simulink model "ur3_simulink_ros2_ibvs_mpc"  (R2023b)
settings: Solver=ode4  StartTime=0.0  StopTime=Inf  FixedStep=0.005  RelTol=1e-3
model workspace (MAT data in the model file):
  SL_ROS_VariableLengthArrays_MaxSizes.CommonInfo.ArrayTruncateAction = 'EmitWarning'
  SL_ROS_VariableLengthArrays_MaxSizes.MsgTypeMap = containers.Map
  SL_ROS_VariableLengthArrays_MaxSizes.MsgTypeMap.serialization.keys = {'example_interfaces/Float64MultiArray'}
  SL_ROS_VariableLengthArrays_MaxSizes.MsgTypeMap.serialization.values{1}.PropertyName = 'data'
  SL_ROS_VariableLengthArrays_MaxSizes.MsgTypeMap.serialization.values{1}.DataType = 'double'
  SL_ROS_VariableLengthArrays_MaxSizes.MsgTypeMap.serialization.values{1}.MaxLength = 1
  SL_ROS_VariableLengthArrays_MaxSizes.MsgTypeMap.serialization.uniformity = 0
  SL_ROS_VariableLengthArrays_MaxSizes.MsgTypeMap.serialization.keyType = 'char'
  SL_ROS_VariableLengthArrays_MaxSizes.MsgTypeMap.serialization.valueType = 'any'
undefined symbols (not defined in the file): data, data_SL_Info
libraries: simulink x9, ros2lib x8, robotmaniplib x3, robotcorelib x2, dspinverses x1, mpclib x1
(part 1 of 2)
settings Model: SimulationMode=accelerator  Creator=81232  LastModifiedBy=Administrator
settings OptimizationCC: EnhancedBackFolding=on  PassReuseOutputArgsAs=Individual arguments  ZeroExternalMemoryAtStartup=off  ZeroInternalMemoryAtStartup=off  MaxStackSize=64  OptimizeBlockOrder=speed  DifferentSizesBufferReuse=on  OptimizationCustomize=off  EfficientTunableParamExpr=on
settings DebuggingCC: ParameterTunabilityLossMsg=error
settings ModelReferenceCC: EnableRefExpFcnMdlSchedulingChecks=on
settings SFSimCC: MATLABDynamicMemAlloc=off
settings RTWCC: Description=Embedded Coder  SystemTargetFile=ert.tlc  HardwareBoard=Robot Operating System 2 (ROS 2)  TLCOptions="-aInlineSetEventsForThisBaseRateFcn=TLC_FALSE -aSuppressMultiTaskScheduler=TLC_FALSE  -aRateBasedStepFcn=0"  TemplateMakefile=ert_default_tmf  Toolchain=Colcon Tools  TargetLang=C++
settings CodeAppCC: ForceParamTrailComments=on  IgnoreCustomStorageClasses=off  OperatorAnnotations=on  SimulinkDataObjDesc=on  SFDataObjDesc=on  InsertBlockDesc=on
settings ERTTargetCC: CodeInterfacePackaging=C++ class  RootIOFormat=Structure reference

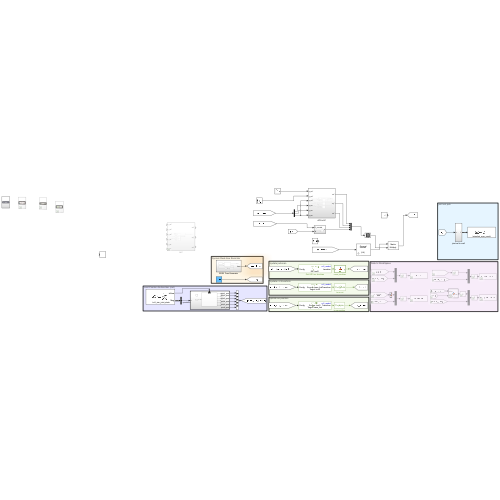
[thumbnail: Simulink's stored preview of the top-level diagram]
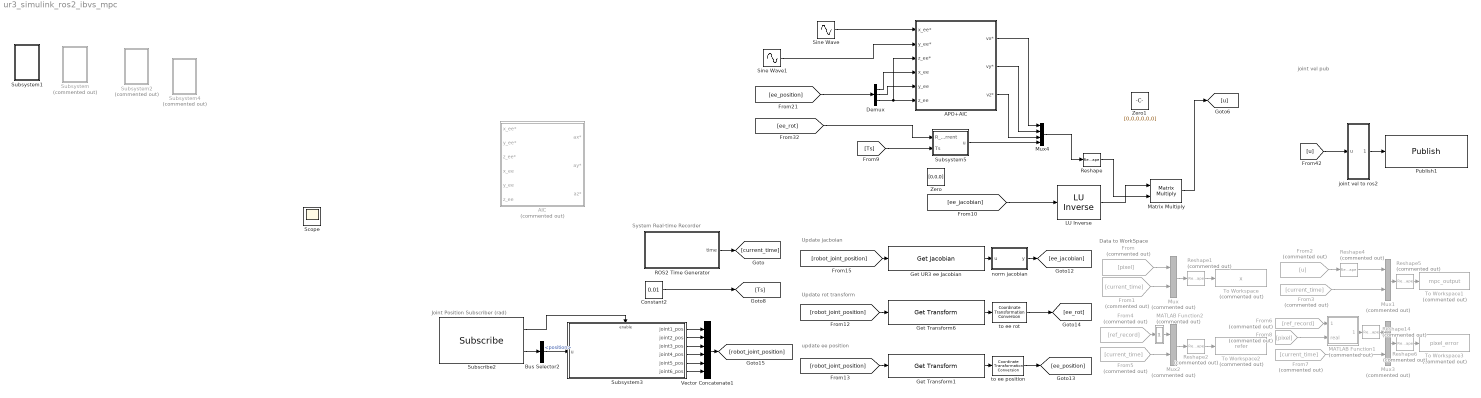
== system ur3_simulink_ros2_ibvs_mpc ==
  note: joint vel pub
  note: update ee position
  note: Update rot transform
  note: Joint Position Subscriber (rad)
  note: Data to WorkSpace
  note: System Real-time Recorder
  note: Update jacboian
  " LU Inverse" : dspinverses/ LU Inverse
  AIC : Subsystem  Commented=on
  APO+AIC : Subsystem
  Bus Selector2 : BusSelector  OutputSignals=position
  Constant2 : Constant  Value=0.01
  Demux : Demux  Outputs=3
  From : From  Commented=on  GotoTag=pixel
  From{1,3,5,7} (4 alike) : From  Commented=on  GotoTag=current_time
  From2 : From  Commented=on  GotoTag=u
  From4 : From  Commented=on  GotoTag=ref_record
  From6 : From  Commented=on  GotoTag=ref_record
  From8 : From  Commented=on  GotoTag=pixel
  Get Transform1 : robotmaniplib/Get Transform  RigidBodyTree=ur3_model  SourceBody=tool0  TargetBody=base_link  SimulateUsing=Interpreted execution
  Get Transform6 : robotmaniplib/Get Transform  RigidBodyTree=ur3_model  SourceBody=base_link  TargetBody=tool0  SimulateUsing=Interpreted execution
  Get UR3 ee Jacobian : robotmaniplib/Get Jacobian  RigidBodyTree=ur3_model  EndEffector=tool0  SimulateUsing=Interpreted execution
  MATLAB Function1 : MATLAB Function  Commented=on  TreatAsAtomicUnit=on
  MATLAB Function2 : MATLAB Function  Commented=on  TreatAsAtomicUnit=on
  Matrix Multiply : Product  Multiplication=Matrix(*)
  Mux{,1..3} (4 alike) : Mux  Commented=on  Inputs=2
  Mux4 : Mux
  Publish1 : ros2lib/Publish  topicSource=Select from ROS network  topic=/simulink_mpc_result  messageType=std_msgs/Float64MultiArray  QOSHistory=Keep last  QOSDepth=1  QOSReliability=Reliable  QOSDurability=Volatile
      settings: LibrarySourceBlock=roslib/ROS 2/Publish
  ROS2 Time Generator : Subsystem
  Reshape : Reshape  OutputDimensionality=Column vector (2-D)
  Reshape1 : Reshape  Commented=on  OutputDimensionality=Customize  OutputDimensions=[9]
  Reshape14 : Reshape  Commented=on  OutputDimensionality=Customize  OutputDimensions=[8,1]
  Reshape2 : Reshape  Commented=on  OutputDimensionality=Customize  OutputDimensions=[9]
  Reshape4 : Reshape  Commented=on  OutputDimensionality=Customize  OutputDimensions=[6,1]
  Reshape5 : Reshape  Commented=on  OutputDimensionality=Customize  OutputDimensions=[7]
  Reshape6 : Reshape  Commented=on  OutputDimensionality=Customize  OutputDimensions=[9]
  Scope : Scope
  Sine Wave : Sin  Amplitude=0.15  Bias=-0.1  Frequency=1.6  SampleTime=0
  Sine Wave1 : Sin  Amplitude=0.15  Bias=0.3  Frequency=1.6  Phase=pi/2  SampleTime=0
  Subscribe2 : ros2lib/Subscribe  topicSource=Select from ROS network  topic=/ur3_sim_joint_state  messageType=sensor_msgs/JointState  sampleTime=0.005  QOSHistory=Keep last  QOSDepth=1  QOSReliability=Reliable  QOSDurability=Volatile
  Subsystem : Subsystem  Commented=on
  Subsystem1 : Subsystem
  Subsystem2 : Subsystem  Commented=on
  Subsystem3 : Subsystem
  Subsystem4 : Subsystem  Commented=on
  Subsystem5 : Subsystem
  To Workspace : ToWorkspace  Commented=on  VariableName=x  SaveFormat=Timeseries  SampleTime=-1
  To Workspace1 : ToWorkspace  Commented=on  VariableName=mpc_output  SaveFormat=Timeseries  SampleTime=-1
  To Workspace2 : ToWorkspace  Commented=on  VariableName=refer  SaveFormat=Timeseries  SampleTime=-1
  To Workspace3 : ToWorkspace  Commented=on  VariableName=pixel_error  SaveFormat=Timeseries  SampleTime=-1
  Vector Concatenate1 : Concatenate  NumInputs=6
  Zero : Constant  Value=[0,0,0]  OutDataTypeStr=Inherit: Inherit via back propagation
  Zero1 : Constant  Value=[0,0,0,0,0,0]  OutDataTypeStr=Inherit: Inherit via back propagation
  joint vel to ros2 : Subsystem
  norm jacobian : MATLAB Function  TreatAsAtomicUnit=on
  to ee position : robotcorelib/Coordinate Transformation Conversion  InputRepresentation=Homogeneous Transformation  InputEulerSequence=ZYX  ShowTrVecInputPort=on  OutputRepresentation=Translation Vector  OutputEulerSequence=ZYX  ShowTrVecOutputPort=off  SimulateUsing=Interpreted execution
  to ee rot : robotcorelib/Coordinate Transformation Conversion  InputRepresentation=Homogeneous Transformation  InputEulerSequence=ZYX  ShowTrVecInputPort=on  OutputRepresentation=Rotation Matrix  OutputEulerSequence=ZYX  ShowTrVecOutputPort=off  SimulateUsing=Interpreted execution
  wires:
  ROS2 Time Generator/1(time) -> [current_time]
  From/1 -> Mux/1
  From1/1 -> Mux/2
  From2/1 -> Reshape4/1
  From3/1 -> Mux1/2
  From5/1 -> Mux2/2
  Mux2/1 -> Reshape2/1
  From7/1 -> Mux3/2
  From6/1 -> MATLAB Function1/1(refer)
  From8/1 -> MATLAB Function1/2(real)
  joint vel to ros2/1(Out1) -> Publish1/1
  Mux3/1 -> Reshape6/1
  MATLAB Function1/1(pixel_error) -> Reshape14/1
  Reshape14/1 -> Mux3/1
  Reshape4/1 -> Mux1/1
  Mux1/1 -> Reshape5/1
  Reshape5/1 -> To Workspace1/1
  Reshape6/1 -> To Workspace3/1
  Subscribe2/2 -> Bus Selector2/1
  Bus Selector2/1 -> Subsystem3/1(u)  "<position>"
  Subscribe2/1 -> Subsystem3/Enable
  Subsystem3/1(joint1_pos) -> Vector Concatenate1/1
  Subsystem3/2(joint2_pos) -> Vector Concatenate1/2
  Subsystem3/3(joint3_pos) -> Vector Concatenate1/3
  Subsystem3/4(joint4_pos) -> Vector Concatenate1/4
  Subsystem3/5(joint5_pos) -> Vector Concatenate1/5
  Subsystem3/6(joint6_pos) -> Vector Concatenate1/6
  norm jacobian/1(y) -> [ee_jacobian]
  Get UR3 ee Jacobian/1 -> norm jacobian/1(u)
  [robot_joint_position] -> Get Transform6/1
  Get Transform6/1 -> to ee rot/1
  to ee rot/1 -> [ee_rot]
  to ee position/1 -> [ee_position]
  Get Transform1/1 -> to ee position/1
  [robot_joint_position] -> Get UR3 ee Jacobian/1
  [robot_joint_position] -> Get Transform1/1
  Vector Concatenate1/1 -> [robot_joint_position]
  [u] -> joint vel to ros2/1(u)
  Mux/1 -> Reshape1/1
  Reshape1/1 -> To Workspace/1
  Reshape2/1 -> To Workspace2/1
  MATLAB Function2/1(y) -> Mux2/1
  From4/1 -> MATLAB Function2/1(u)
  Constant2/1 -> [Ts]
  [ee_position] -> Demux/1
  [Ts] -> Subsystem5/2(Ts)
  Demux/1 -> APO+AIC/4(x_ee)
  Demux/2 -> APO+AIC/5(y_ee)
  Demux/3 -> APO+AIC/3(z_ee*), APO+AIC/6(z_ee)
  Sine Wave/1 -> APO+AIC/1(x_ee*)
  APO+AIC/1(vx*) -> Mux4/1
  APO+AIC/2(vy*) -> Mux4/2
  Mux4/1 -> Reshape/1
  [ee_jacobian] -> " LU Inverse"/1
  " LU Inverse"/1 -> Matrix Multiply/1
  Reshape/1 -> Matrix Multiply/2
  Sine Wave1/1 -> APO+AIC/2(y_ee*)
  Matrix Multiply/1 -> [u]
  [ee_rot] -> Subsystem5/1(R_current)
  APO+AIC/3(vz*) -> Mux4/3
  Subsystem5/1(u) -> Mux4/4

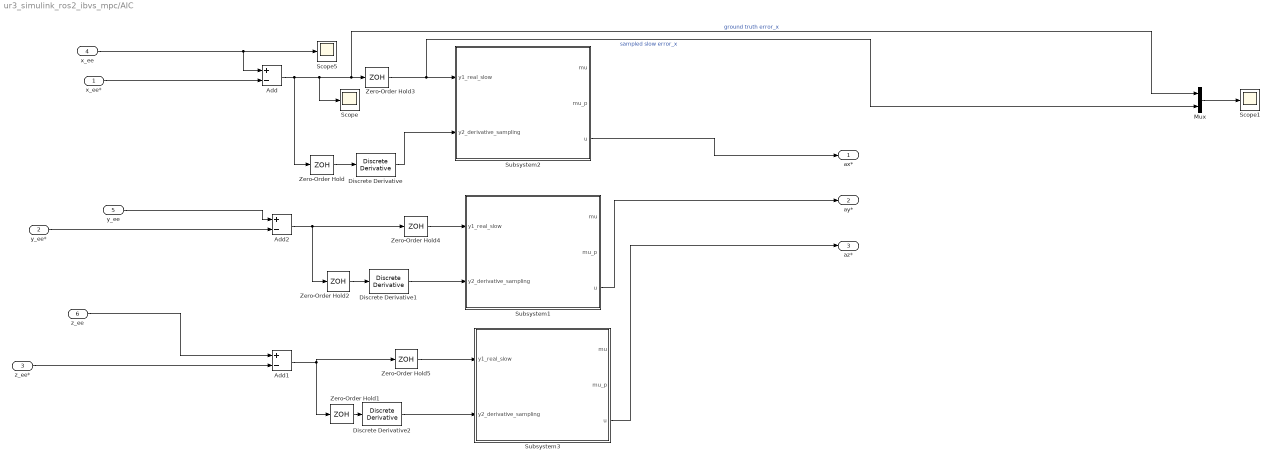
== system ur3_simulink_ros2_ibvs_mpc/AIC ==
  x_ee* : Inport
  y_ee* : Inport  Port=2
  z_ee* : Inport  Port=3
  x_ee : Inport  Port=4
  y_ee : Inport  Port=5
  z_ee : Inport  Port=6
  Add : Sum  Inputs=+-
  Add1 : Sum  Inputs=+-
  Add2 : Sum  Inputs=+-
  Discrete Derivative : simulink/Discrete/Discrete Derivative  gainval=1.0  ICPrevScaledInput=0.0  OutMin=[]  OutMax=[]  OutDataType=fixdt(1, 16)  OutScaling=2^-10  DoSatur=off
  Discrete Derivative1 : simulink/Discrete/Discrete Derivative  gainval=1.0  ICPrevScaledInput=0.0  OutMin=[]  OutMax=[]  OutDataType=fixdt(1, 16)  OutScaling=2^-10  DoSatur=off
  Discrete Derivative2 : simulink/Discrete/Discrete Derivative  gainval=1.0  ICPrevScaledInput=0.0  OutMin=[]  OutMax=[]  OutDataType=fixdt(1, 16)  OutScaling=2^-10  DoSatur=off
  Mux : Mux  Inputs=2
  Scope : Scope
  Scope1 : Scope
  Scope5 : Scope
  Subsystem1 : Subsystem
  Subsystem2 : Subsystem
  Subsystem3 : Subsystem
  Zero-Order Hold{,1..5} (6 alike) : ZeroOrderHold  SampleTime=0.05
  ax* : Outport
  ay* : Outport  Port=2
  az* : Outport  Port=3
  wires:
  Add2/1 -> Zero-Order Hold4/1, Zero-Order Hold2/1
  x_ee/1 -> Add/1, Scope5/1
  Discrete Derivative/1 -> Subsystem2/2(y2_derivative_sampling)
  Zero-Order Hold/1 -> Discrete Derivative/1
  Add1/1 -> Zero-Order Hold5/1, Zero-Order Hold1/1
  x_ee*/1 -> Add/2
  y_ee/1 -> Add2/1
  z_ee/1 -> Add1/1
  Subsystem3/3(u) -> az*/1
  Zero-Order Hold1/1 -> Discrete Derivative2/1
  Zero-Order Hold2/1 -> Discrete Derivative1/1
  y_ee*/1 -> Add2/2
  Discrete Derivative2/1 -> Subsystem3/2(y2_derivative_sampling)
  Subsystem1/3(u) -> ay*/1
  z_ee*/1 -> Add1/2
  Discrete Derivative1/1 -> Subsystem1/2(y2_derivative_sampling)
  Subsystem2/3(u) -> ax*/1
  Zero-Order Hold4/1 -> Subsystem1/1(y1_real_slow)
  Zero-Order Hold5/1 -> Subsystem3/1(y1_real_slow)
  Zero-Order Hold3/1 -> Mux/2, Subsystem2/1(y1_real_slow)  "sampled slow error_x"
  Mux/1 -> Scope1/1
  Add/1 -> Zero-Order Hold/1, Scope/1, Mux/1, Zero-Order Hold3/1  "ground truth error_x"

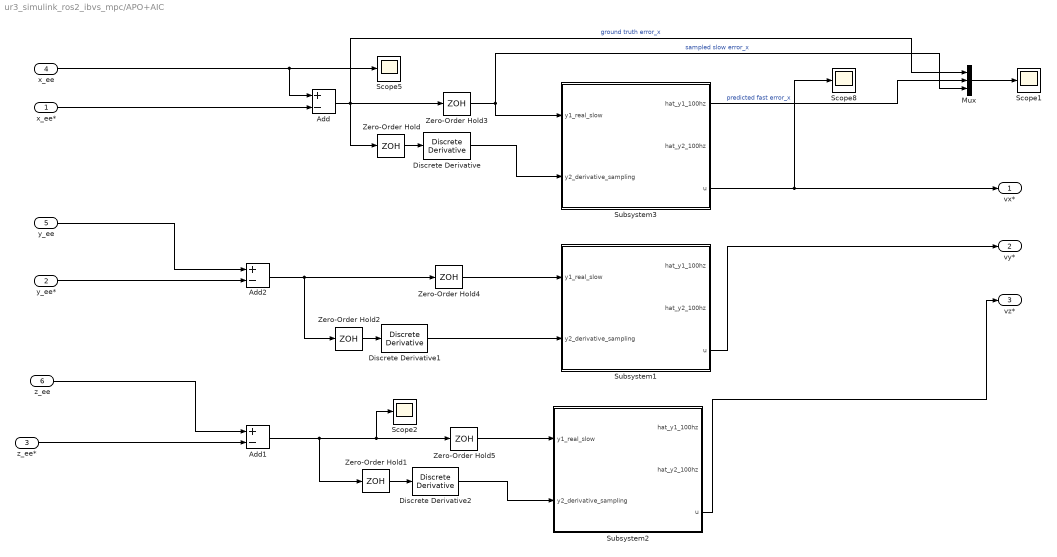
== system ur3_simulink_ros2_ibvs_mpc/APO+AIC ==
  x_ee* : Inport
  y_ee* : Inport  Port=2
  z_ee* : Inport  Port=3
  x_ee : Inport  Port=4
  y_ee : Inport  Port=5
  z_ee : Inport  Port=6
  Add : Sum  Inputs=+-
  Add1 : Sum  Inputs=+-
  Add2 : Sum  Inputs=+-
  Discrete Derivative : simulink/Discrete/Discrete Derivative  gainval=1.0  ICPrevScaledInput=0  OutMin=[]  OutMax=[]  OutDataType=fixdt(1, 16)  OutScaling=2^-10  DoSatur=off
  Discrete Derivative1 : simulink/Discrete/Discrete Derivative  gainval=1.0  ICPrevScaledInput=0.0  OutMin=[]  OutMax=[]  OutDataType=fixdt(1, 16)  OutScaling=2^-10  DoSatur=off
  Discrete Derivative2 : simulink/Discrete/Discrete Derivative  gainval=1.0  ICPrevScaledInput=0.0  OutMin=[]  OutMax=[]  OutDataType=fixdt(1, 16)  OutScaling=2^-10  DoSatur=off
  Mux : Mux  Inputs=3
  Scope{1..2,5,8} (4 alike) : Scope
  Subsystem1 : Subsystem
  Subsystem2 : Subsystem
  Subsystem3 : Subsystem
  Zero-Order Hold{,1..5} (6 alike) : ZeroOrderHold  SampleTime=0.05
  vx* : Outport
  vy* : Outport  Port=2
  vz* : Outport  Port=3
  wires:
  Add2/1 -> Zero-Order Hold4/1, Zero-Order Hold2/1
  x_ee/1 -> Add/1, Scope5/1
  Discrete Derivative/1 -> Subsystem3/2(y2_derivative_sampling)
  Zero-Order Hold/1 -> Discrete Derivative/1
  Discrete Derivative1/1 -> Subsystem1/2(y2_derivative_sampling)
  Add1/1 -> Zero-Order Hold5/1, Scope2/1, Zero-Order Hold1/1
  Subsystem3/3(u) -> vx*/1, Scope8/1
  Add/1 -> Mux/1, Zero-Order Hold/1, Zero-Order Hold3/1  "ground truth error_x"
  x_ee*/1 -> Add/2
  y_ee/1 -> Add2/1
  z_ee/1 -> Add1/1
  Subsystem2/3(u) -> vz*/1
  Zero-Order Hold1/1 -> Discrete Derivative2/1
  Zero-Order Hold2/1 -> Discrete Derivative1/1
  y_ee*/1 -> Add2/2
  z_ee*/1 -> Add1/2
  Zero-Order Hold3/1 -> Mux/3, Subsystem3/1(y1_real_slow)  "sampled slow error_x"
  Zero-Order Hold4/1 -> Subsystem1/1(y1_real_slow)
  Zero-Order Hold5/1 -> Subsystem2/1(y1_real_slow)
  Subsystem1/3(u) -> vy*/1
  Subsystem3/1(hat_y1_100hz) -> Mux/2  "predicted fast error_x"
  Mux/1 -> Scope1/1
  Discrete Derivative2/1 -> Subsystem2/2(y2_derivative_sampling)

== system ur3_simulink_ros2_ibvs_mpc/ROS2 Time Generator ==
  Current Time : ros2lib/Current Time  OutputFormat=double  SampleTime=0.005  ModelName=ur3_simulink_ros2_ibvs_mpc
      settings: LibrarySourceBlock=roslib/ROS 2/Current Time
  Current Time1 : ros2lib/Current Time  OutputFormat=double  SampleTime=0.005  ModelName=ur3_simulink_ros2_ibvs_mpc
      settings: LibrarySourceBlock=roslib/ROS 2/Current Time
  Delay : Delay  DelayLength=1  InitialConditionSource=Input port
      settings: InputPortMap=u0,p4
  MATLAB Function : MATLAB Function  TreatAsAtomicUnit=on
  time : Outport
  wires:
  Delay/1 -> MATLAB Function/2(last_time)
  Current Time1/1 -> Delay/2
  MATLAB Function/2(init_time) -> Delay/1
  Current Time/1 -> MATLAB Function/1(current_time)
  MATLAB Function/1(time_x) -> time/1

== system ur3_simulink_ros2_ibvs_mpc/Subsystem ==
  note: Refer Publihser
  Blank Message : ros2lib/Blank Message  messageClass=Message  entityType=std_msgs/Float64MultiArray  messageType=std_msgs/Float64MultiArray  SampleTime=inf
      settings: LibrarySourceBlock=roslib/ROS 2/Blank Message
  Bus Assignment : BusAssignment  AssignedSignals=data
  Constant1 : Constant  Value=75
  MATLAB Function : MATLAB Function  TreatAsAtomicUnit=on
  Publish : ros2lib/Publish  topicSource=Specify your own  topic=/image_refer  messageType=std_msgs/Float64MultiArray  QOSHistory=Keep last  QOSDepth=1  QOSReliability=Reliable  QOSDurability=Volatile
      settings: LibrarySourceBlock=roslib/ROS 2/Publish
  wires:
  MATLAB Function/1(y) -> Bus Assignment/2
  Blank Message/1 -> Bus Assignment/1
  Constant1/1 -> [refer], MATLAB Function/1(u)
  Bus Assignment/1 -> Publish/1

== system ur3_simulink_ros2_ibvs_mpc/Subsystem1 ==
  note: Image Pixel Subscriber
  Bus Selector : BusSelector  Commented=on  OutputSignals=data
  Goto1 : Goto  Commented=on  GotoTag=pixel
  Subscribe : ros2lib/Subscribe  Commented=on  topicSource=Select from ROS network  topic=/current_pixel  messageType=std_msgs/Float64MultiArray  sampleTime=-1  QOSHistory=Keep last  QOSDepth=1  QOSReliability=Reliable  QOSDurability=Volatile
  Subsystem : Subsystem  Commented=on
  wires:
  Subscribe/2 -> Bus Selector/1
  Subsystem/1(X_in) -> Goto1/1
  Subscribe/1 -> Subsystem/Enable
  Bus Selector/1 -> Subsystem/1(u)  "<data>"

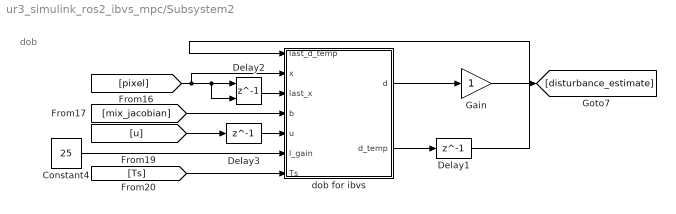
== system ur3_simulink_ros2_ibvs_mpc/Subsystem2 ==
  note: dob
  Constant4 : Constant  Value=25
  Delay1 : Delay  DelayLength=1
  Delay2 : Delay  DelayLength=1  InitialConditionSource=Input port
      settings: InputPortMap=u0,p4
  Delay3 : Delay  DelayLength=1
  Gain : Gain
  dob for ibvs : MATLAB Function  TreatAsAtomicUnit=on
  wires:
  dob for ibvs/2(d_temp) -> Delay1/1
  Delay2/1 -> dob for ibvs/3(last_x)
  [u] -> Delay3/1
  Delay1/1 -> dob for ibvs/1(last_d_temp)
  [Ts] -> dob for ibvs/7(Ts)
  [mix_jacobian] -> dob for ibvs/4(b)
  Constant4/1 -> dob for ibvs/6(l_gain)
  dob for ibvs/1(d) -> Gain/1
  Gain/1 -> [disturbance_estimate]
  [pixel] -> Delay2/2, Delay2/1, dob for ibvs/2(x)
  Delay3/1 -> dob for ibvs/5(u)

== system ur3_simulink_ros2_ibvs_mpc/Subsystem3 ==
  u : Inport
  Enable : EnablePort
  MATLAB Function : MATLAB Function  TreatAsAtomicUnit=on
  joint1_pos : Outport
  joint2_pos : Outport  Port=2
  joint3_pos : Outport  Port=3
  joint4_pos : Outport  Port=4
  joint5_pos : Outport  Port=5
  joint6_pos : Outport  Port=6
  wires:
  u/1 -> MATLAB Function/1(u)
  MATLAB Function/1(joint1_pos) -> joint1_pos/1
  MATLAB Function/2(joint2_pos) -> joint2_pos/1
  MATLAB Function/3(joint3_pos) -> joint3_pos/1
  MATLAB Function/4(joint4_pos) -> joint4_pos/1
  MATLAB Function/5(joint5_pos) -> joint5_pos/1
  MATLAB Function/6(joint6_pos) -> joint6_pos/1

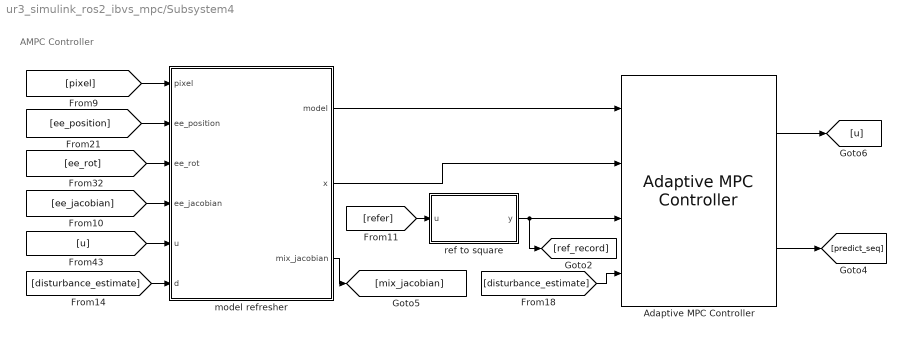
== system ur3_simulink_ros2_ibvs_mpc/Subsystem4 ==
  note: AMPC Controller
  Adaptive MPC Controller : mpclib/Adaptive MPC Controller  SCDEnableBlockLinearizationSpecification=on  mpcobj=mpcobj  enable_value=0  updateMPCinCallerWorkspace=on  md_inport=on  mv_inport=off  uref_inport=off  return_cost=off  return_mvseq=off  return_qpstatus=off  return_xseq=on  return_state=off  return_ovseq=off  state_inport=on  isltv_plant=off  umin_inport=off  umax_inport=off  ymin_inport=off  ymax_inport=off  cc_inport=off  ywt_inport=off  uwt_inport=off  duwt_inport=off  rhoeps_inport=off  pm_inport=off  MaximumP=10  HorizonChoice=FixedHorizon  BlockDataType=double  SampleTimeInherited=off  switch_inport=off
  model refresher : Subsystem
  ref to square : MATLAB Function  TreatAsAtomicUnit=on
  wires:
  [ee_rot] -> model refresher/3(ee_rot)
  [ee_jacobian] -> model refresher/4(ee_jacobian)
  model refresher/2(x) -> Adaptive MPC Controller/2
  ref to square/1(y) -> Adaptive MPC Controller/3, [ref_record]
  [pixel] -> model refresher/1(pixel)
  [refer] -> ref to square/1(u)
  model refresher/1(model) -> Adaptive MPC Controller/1
  Adaptive MPC Controller/2 -> [predict_seq]
  model refresher/3(mix_jacobian) -> [mix_jacobian]
  [ee_position] -> model refresher/2(ee_position)
  [u] -> model refresher/5(u)
  [disturbance_estimate] -> model refresher/6(d)
  Adaptive MPC Controller/1 -> [u]
  [disturbance_estimate] -> Adaptive MPC Controller/4

== system ur3_simulink_ros2_ibvs_mpc/Subsystem5 ==
  R_current : Inport
  Ts : Inport  Port=2
  Discrete Pulse Generator : DiscretePulseGenerator  SampleTime=0.005
  attitude_pi_ctrl : Subsystem
  u : Outport
  wires:
  Ts/1 -> attitude_pi_ctrl/2(Ts)
  Discrete Pulse Generator/1 -> attitude_pi_ctrl/Trigger
  R_current/1 -> attitude_pi_ctrl/1(R_current)
  attitude_pi_ctrl/1(u) -> u/1

== system ur3_simulink_ros2_ibvs_mpc/joint vel to ros2 ==
  u : Inport
  Blank Message1 : ros2lib/Blank Message  messageClass=Message  entityType=std_msgs/Float64MultiArray  messageType=std_msgs/Float64MultiArray  SampleTime=inf
      settings: LibrarySourceBlock=roslib/ROS 2/Blank Message
  Bus Assignment1 : BusAssignment  AssignedSignals=data,data_SL_Info.CurrentLength,data_SL_Info.ReceivedLength
  Constant : Constant  Value=128  OutDataTypeStr=uint32
  Constant2 : Constant  Value=128  OutDataTypeStr=uint32
  to ros2 : MATLAB Function  TreatAsAtomicUnit=on
  Out1 : Outport
  wires:
  u/1 -> to ros2/1(u)
  to ros2/1(y) -> Bus Assignment1/2
  Constant2/1 -> Bus Assignment1/4
  Constant/1 -> Bus Assignment1/3
  Blank Message1/1 -> Bus Assignment1/1
  Bus Assignment1/1 -> Out1/1

== system ur3_simulink_ros2_ibvs_mpc/AIC/Subsystem1 ==
  y1_real_slow : Inport
  y2_derivative_sampling : Inport  Port=2
  AIC_muti_sensor_module : Subsystem
  Discrete Pulse Generator : DiscretePulseGenerator  Period=10  SampleTime=0.005
  mu : Outport
  mu_p : Outport  Port=2
  u : Outport  Port=3
  wires:
  AIC_muti_sensor_module/1(u) -> u/1  "u"
  y1_real_slow/1 -> AIC_muti_sensor_module/1(y1_real_slow)
  y2_derivative_sampling/1 -> AIC_muti_sensor_module/2(y2_derivative_sampling)
  Discrete Pulse Generator/1 -> AIC_muti_sensor_module/Trigger
  AIC_muti_sensor_module/3(mu_p) -> mu_p/1
  AIC_muti_sensor_module/2(mu) -> mu/1

== system ur3_simulink_ros2_ibvs_mpc/AIC/Subsystem2 ==
  y1_real_slow : Inport
  y2_derivative_sampling : Inport  Port=2
  AIC_muti_sensor_module : Subsystem
  Discrete Pulse Generator : DiscretePulseGenerator  Period=10  SampleTime=0.005
  mu : Outport
  mu_p : Outport  Port=2
  u : Outport  Port=3
  wires:
  AIC_muti_sensor_module/1(u) -> u/1  "u"
  y1_real_slow/1 -> AIC_muti_sensor_module/1(y1_real_slow)
  y2_derivative_sampling/1 -> AIC_muti_sensor_module/2(y2_derivative_sampling)
  Discrete Pulse Generator/1 -> AIC_muti_sensor_module/Trigger
  AIC_muti_sensor_module/3(mu_p) -> mu_p/1
  AIC_muti_sensor_module/2(mu) -> mu/1

== system ur3_simulink_ros2_ibvs_mpc/AIC/Subsystem3 ==
  y1_real_slow : Inport
  y2_derivative_sampling : Inport  Port=2
  AIC_muti_sensor_module : Subsystem
  Discrete Pulse Generator : DiscretePulseGenerator  Period=10  SampleTime=0.005
  mu : Outport
  mu_p : Outport  Port=2
  u : Outport  Port=3
  wires:
  AIC_muti_sensor_module/1(u) -> u/1  "u"
  y1_real_slow/1 -> AIC_muti_sensor_module/1(y1_real_slow)
  y2_derivative_sampling/1 -> AIC_muti_sensor_module/2(y2_derivative_sampling)
  Discrete Pulse Generator/1 -> AIC_muti_sensor_module/Trigger
  AIC_muti_sensor_module/3(mu_p) -> mu_p/1
  AIC_muti_sensor_module/2(mu) -> mu/1

== system ur3_simulink_ros2_ibvs_mpc/APO+AIC/Subsystem1 ==
  y1_real_slow : Inport
  y2_derivative_sampling : Inport  Port=2
  APO+AIC : Subsystem
  Discrete Pulse Generator1 : DiscretePulseGenerator  SampleTime=0.005
  Selector : Selector  InputPortWidth=2  IndexOptions=Index vector (dialog)  Indices=[1]  OutputSizes=1
  Selector1 : Selector  InputPortWidth=2  IndexOptions=Index vector (dialog)  Indices=[2]  OutputSizes=1
  hat_y1_100hz : Outport
  hat_y2_100hz : Outport  Port=2
  u : Outport  Port=3
  wires:
  y1_real_slow/1 -> APO+AIC/1(y1_real_slow)
  y2_derivative_sampling/1 -> APO+AIC/2(y2_real_slow)
  Selector1/1 -> hat_y2_100hz/1
  Discrete Pulse Generator1/1 -> APO+AIC/Trigger
  APO+AIC/1(hat_x) -> Selector/1, Selector1/1
  Selector/1 -> hat_y1_100hz/1
  APO+AIC/2(u) -> u/1

== system ur3_simulink_ros2_ibvs_mpc/APO+AIC/Subsystem2 ==
  y1_real_slow : Inport
  y2_derivative_sampling : Inport  Port=2
  APO+AIC : Subsystem
  Discrete Pulse Generator1 : DiscretePulseGenerator  SampleTime=0.005
  Selector : Selector  InputPortWidth=2  IndexOptions=Index vector (dialog)  Indices=[1]  OutputSizes=1
  Selector1 : Selector  InputPortWidth=2  IndexOptions=Index vector (dialog)  Indices=[2]  OutputSizes=1
  hat_y1_100hz : Outport
  hat_y2_100hz : Outport  Port=2
  u : Outport  Port=3
  wires:
  y1_real_slow/1 -> APO+AIC/1(y1_real_slow)
  y2_derivative_sampling/1 -> APO+AIC/2(y2_real_slow)
  Selector1/1 -> hat_y2_100hz/1
  Discrete Pulse Generator1/1 -> APO+AIC/Trigger
  APO+AIC/1(hat_x) -> Selector/1, Selector1/1
  Selector/1 -> hat_y1_100hz/1
  APO+AIC/2(u) -> u/1

== system ur3_simulink_ros2_ibvs_mpc/APO+AIC/Subsystem3 ==
  y1_real_slow : Inport
  y2_derivative_sampling : Inport  Port=2
  APO+AIC : Subsystem
  Discrete Pulse Generator1 : DiscretePulseGenerator  SampleTime=0.005
  Selector : Selector  InputPortWidth=2  IndexOptions=Index vector (dialog)  Indices=[1]  OutputSizes=1
  Selector1 : Selector  InputPortWidth=2  IndexOptions=Index vector (dialog)  Indices=[2]  OutputSizes=1
  hat_y1_100hz : Outport
  hat_y2_100hz : Outport  Port=2
  u : Outport  Port=3
  wires:
  y1_real_slow/1 -> APO+AIC/1(y1_real_slow)
  y2_derivative_sampling/1 -> APO+AIC/2(y2_real_slow)
  Selector1/1 -> hat_y2_100hz/1
  Discrete Pulse Generator1/1 -> APO+AIC/Trigger
  APO+AIC/1(hat_x) -> Selector/1, Selector1/1
  Selector/1 -> hat_y1_100hz/1
  APO+AIC/2(u) -> u/1

== system ur3_simulink_ros2_ibvs_mpc/Subsystem1/Subsystem ==
  u : Inport
  Enable : EnablePort
  Bus Creator2 : BusCreator  Inputs=8
  MATLAB Function : MATLAB Function  TreatAsAtomicUnit=on
  X_in : Outport
  wires:
  MATLAB Function/2(v1) -> Bus Creator2/2
  MATLAB Function/5(u3) -> Bus Creator2/5
  MATLAB Function/1(u1) -> Bus Creator2/1
  MATLAB Function/4(v2) -> Bus Creator2/4
  MATLAB Function/3(u2) -> Bus Creator2/3
  u/1 -> MATLAB Function/1(u)
  Bus Creator2/1 -> X_in/1
  MATLAB Function/6(v3) -> Bus Creator2/6
  MATLAB Function/7(u4) -> Bus Creator2/7
  MATLAB Function/8(v4) -> Bus Creator2/8

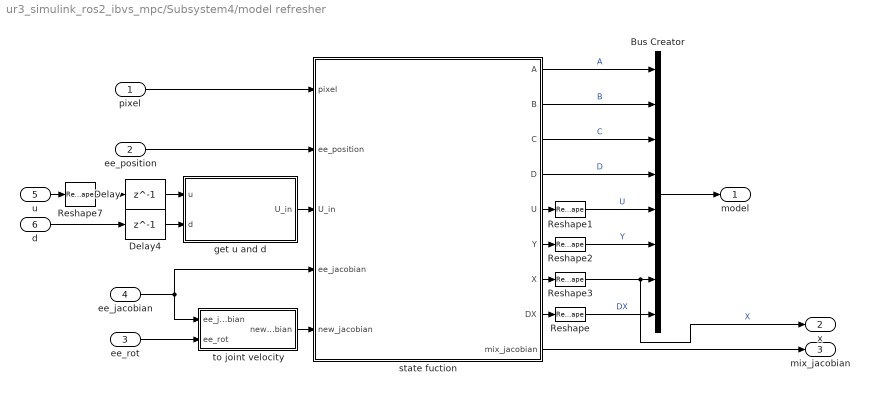
== system ur3_simulink_ros2_ibvs_mpc/Subsystem4/model refresher ==
  pixel : Inport
  ee_position : Inport  Port=2
  ee_rot : Inport  Port=3
  ee_jacobian : Inport  Port=4
  u : Inport  Port=5
  d : Inport  Port=6
  Bus Creator : BusCreator  Inputs=8
  Delay : Delay  DelayLength=1
  Delay4 : Delay  DelayLength=1
  Reshape : Reshape  OutputDimensionality=Customize  OutputDimensions=[11,1]
  Reshape1 : Reshape  OutputDimensionality=Customize  OutputDimensions=[17,1]
  Reshape2 : Reshape  OutputDimensionality=Customize  OutputDimensions=[11,1]
  Reshape3 : Reshape  OutputDimensionality=Customize  OutputDimensions=[11,1]
  Reshape7 : Reshape  OutputDimensionality=Customize  OutputDimensions=[6]
  get u and d : Subsystem
  state fuction : MATLAB Function  TreatAsAtomicUnit=on
  to joint velocity : MATLAB Function  TreatAsAtomicUnit=on
  model : Outport
  x : Outport  Port=2
  mix_jacobian : Outport  Port=3
  wires:
  state fuction/2(B) -> Bus Creator/2  "B"
  state fuction/5(U) -> Reshape1/1
  ee_jacobian/1 -> to joint velocity/1(ee_jacobian), state fuction/4(ee_jacobian)
  pixel/1 -> state fuction/1(pixel)
  state fuction/1(A) -> Bus Creator/1  "A"
  state fuction/4(D) -> Bus Creator/4  "D"
  ee_rot/1 -> to joint velocity/2(ee_rot)
  state fuction/3(C) -> Bus Creator/3  "C"
  ee_position/1 -> state fuction/2(ee_position)
  get u and d/1(U_in) -> state fuction/3(U_in)
  to joint velocity/1(new_jacobian) -> state fuction/5(new_jacobian)
  state fuction/6(Y) -> Reshape2/1
  state fuction/7(X) -> Reshape3/1
  state fuction/8(DX) -> Reshape/1
  state fuction/9(mix_jacobian) -> mix_jacobian/1
  Reshape1/1 -> Bus Creator/5  "U"
  Reshape2/1 -> Bus Creator/6  "Y"
  Reshape3/1 -> x/1, Bus Creator/7  "X"
  Reshape/1 -> Bus Creator/8  "DX"
  Bus Creator/1 -> model/1
  Reshape7/1 -> Delay/1
  Delay4/1 -> get u and d/2(d)
  Delay/1 -> get u and d/1(u)
  u/1 -> Reshape7/1
  d/1 -> Delay4/1

== system ur3_simulink_ros2_ibvs_mpc/Subsystem5/attitude_pi_ctrl ==
  R_current : Inport
  Ts : Inport  Port=2
  Trigger : TriggerPort  VariantControl=(inherit)  PortDimensions=1
  Subsystem : Subsystem
  u : Outport
  wires:
  R_current/1 -> Subsystem/1(R_current)
  Ts/1 -> Subsystem/2(Ts)
  Subsystem/1(u) -> u/1

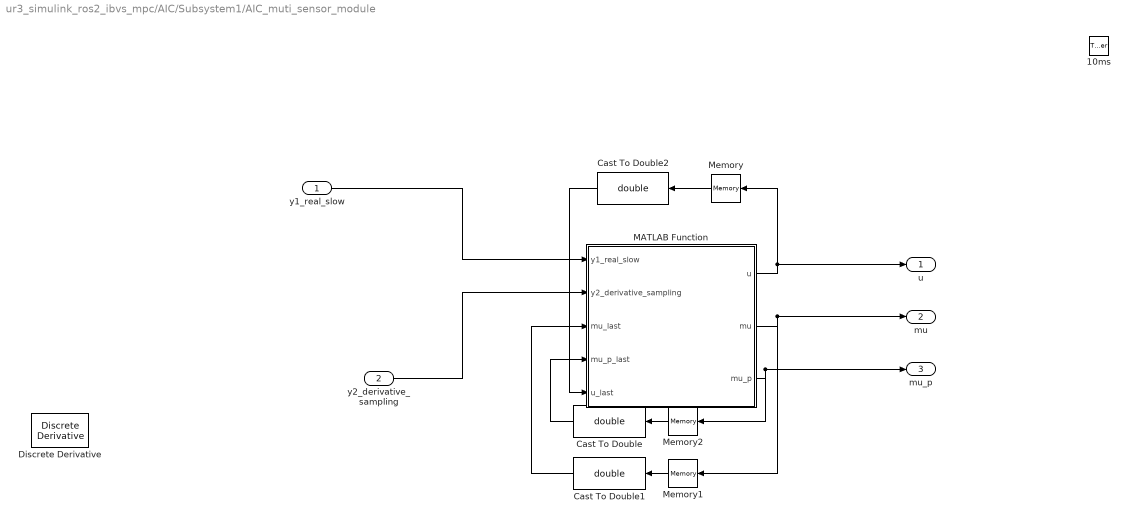
== system ur3_simulink_ros2_ibvs_mpc/AIC/Subsystem1/AIC_muti_sensor_module ==
  y1_real_slow : Inport
  y2_derivative_sampling : Inport  Port=2
  10ms : TriggerPort  VariantControl=(inherit)  InitialTriggerSignalState=zero  PortDimensions=1
  Cast To Double : DataTypeConversion  OutDataTypeStr=double  SaturateOnIntegerOverflow=off  RndMeth=Floor
  Cast To Double1 : DataTypeConversion  OutDataTypeStr=double  SaturateOnIntegerOverflow=off  RndMeth=Floor
  Cast To Double2 : DataTypeConversion  OutDataTypeStr=double  SaturateOnIntegerOverflow=off  RndMeth=Floor
  Discrete Derivative : simulink/Discrete/Discrete Derivative  gainval=1.0  ICPrevScaledInput=0.0  OutMin=[]  OutMax=[]  OutDataType=fixdt(1, 16)  OutScaling=2^-10  DoSatur=off
  MATLAB Function : MATLAB Function  TreatAsAtomicUnit=on
  Memory : Memory  InheritSampleTime=on
  Memory1 : Memory  InheritSampleTime=on
  Memory2 : Memory  InheritSampleTime=on
  u : Outport
  mu : Outport  Port=2
  mu_p : Outport  Port=3
  wires:
  Memory2/1 -> Cast To Double/1
  Memory/1 -> Cast To Double2/1
  y1_real_slow/1 -> MATLAB Function/1(y1_real_slow)
  MATLAB Function/1(u) -> Memory/1, u/1
  MATLAB Function/3(mu_p) -> Memory2/1, mu_p/1
  Memory1/1 -> Cast To Double1/1
  MATLAB Function/2(mu) -> Memory1/1, mu/1
  Cast To Double/1 -> MATLAB Function/4(mu_p_last)
  Cast To Double1/1 -> MATLAB Function/3(mu_last)
  Cast To Double2/1 -> MATLAB Function/5(u_last)
  y2_derivative_sampling/1 -> MATLAB Function/2(y2_derivative_sampling)

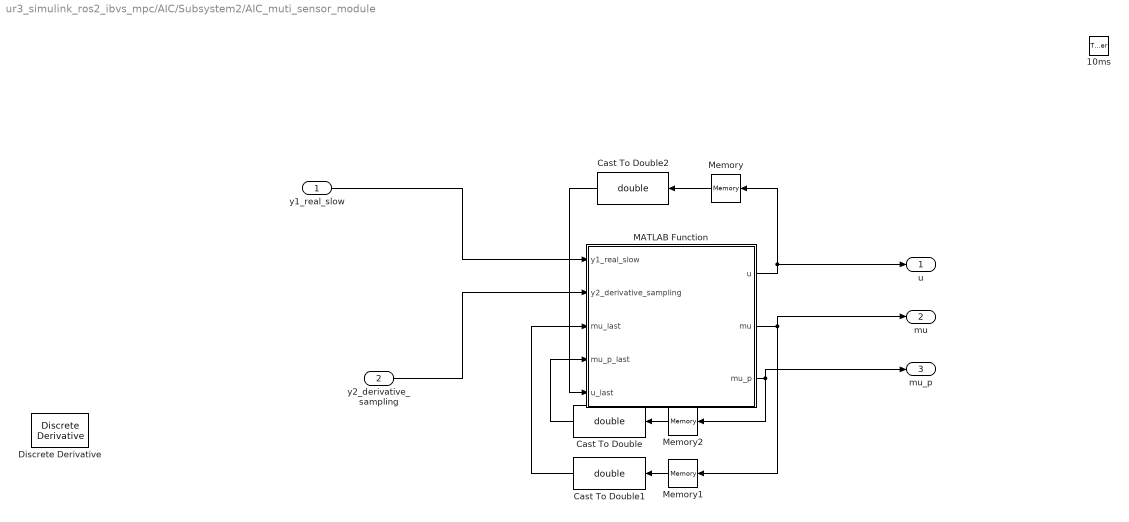
== system ur3_simulink_ros2_ibvs_mpc/AIC/Subsystem2/AIC_muti_sensor_module ==
  y1_real_slow : Inport
  y2_derivative_sampling : Inport  Port=2
  10ms : TriggerPort  VariantControl=(inherit)  InitialTriggerSignalState=zero  PortDimensions=1
  Cast To Double : DataTypeConversion  OutDataTypeStr=double  SaturateOnIntegerOverflow=off  RndMeth=Floor
  Cast To Double1 : DataTypeConversion  OutDataTypeStr=double  SaturateOnIntegerOverflow=off  RndMeth=Floor
  Cast To Double2 : DataTypeConversion  OutDataTypeStr=double  SaturateOnIntegerOverflow=off  RndMeth=Floor
  Discrete Derivative : simulink/Discrete/Discrete Derivative  gainval=1.0  ICPrevScaledInput=0.0  OutMin=[]  OutMax=[]  OutDataType=fixdt(1, 16)  OutScaling=2^-10  DoSatur=off
  MATLAB Function : MATLAB Function  TreatAsAtomicUnit=on
  Memory : Memory  InheritSampleTime=on
  Memory1 : Memory  InheritSampleTime=on
  Memory2 : Memory  InheritSampleTime=on
  u : Outport
  mu : Outport  Port=2
  mu_p : Outport  Port=3
  wires:
  Memory2/1 -> Cast To Double/1
  Memory/1 -> Cast To Double2/1
  y1_real_slow/1 -> MATLAB Function/1(y1_real_slow)
  MATLAB Function/1(u) -> Memory/1, u/1
  MATLAB Function/3(mu_p) -> mu_p/1, Memory2/1
  Memory1/1 -> Cast To Double1/1
  MATLAB Function/2(mu) -> mu/1, Memory1/1
  Cast To Double/1 -> MATLAB Function/4(mu_p_last)
  Cast To Double1/1 -> MATLAB Function/3(mu_last)
  Cast To Double2/1 -> MATLAB Function/5(u_last)
  y2_derivative_sampling/1 -> MATLAB Function/2(y2_derivative_sampling)

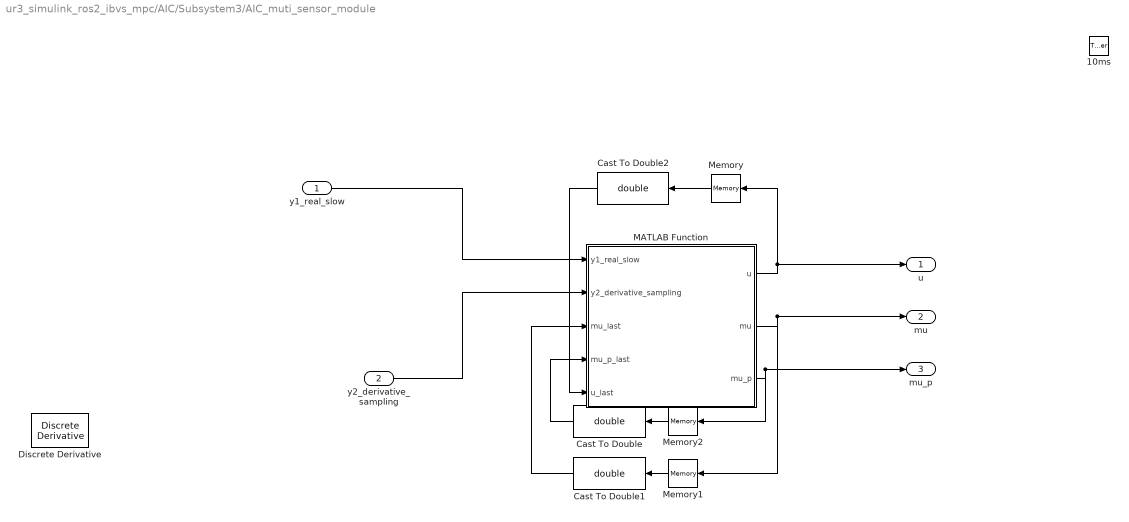
== system ur3_simulink_ros2_ibvs_mpc/AIC/Subsystem3/AIC_muti_sensor_module ==
  y1_real_slow : Inport
  y2_derivative_sampling : Inport  Port=2
  10ms : TriggerPort  VariantControl=(inherit)  InitialTriggerSignalState=zero  PortDimensions=1
  Cast To Double : DataTypeConversion  OutDataTypeStr=double  SaturateOnIntegerOverflow=off  RndMeth=Floor
  Cast To Double1 : DataTypeConversion  OutDataTypeStr=double  SaturateOnIntegerOverflow=off  RndMeth=Floor
  Cast To Double2 : DataTypeConversion  OutDataTypeStr=double  SaturateOnIntegerOverflow=off  RndMeth=Floor
  Discrete Derivative : simulink/Discrete/Discrete Derivative  gainval=1.0  ICPrevScaledInput=0.0  OutMin=[]  OutMax=[]  OutDataType=fixdt(1, 16)  OutScaling=2^-10  DoSatur=off
  MATLAB Function : MATLAB Function  TreatAsAtomicUnit=on
  Memory : Memory  InheritSampleTime=on
  Memory1 : Memory  InheritSampleTime=on
  Memory2 : Memory  InheritSampleTime=on
  u : Outport
  mu : Outport  Port=2
  mu_p : Outport  Port=3
  wires:
  Memory2/1 -> Cast To Double/1
  Memory/1 -> Cast To Double2/1
  y1_real_slow/1 -> MATLAB Function/1(y1_real_slow)
  MATLAB Function/1(u) -> Memory/1, u/1
  MATLAB Function/3(mu_p) -> Memory2/1, mu_p/1
  Memory1/1 -> Cast To Double1/1
  MATLAB Function/2(mu) -> Memory1/1, mu/1
  Cast To Double/1 -> MATLAB Function/4(mu_p_last)
  Cast To Double1/1 -> MATLAB Function/3(mu_last)
  Cast To Double2/1 -> MATLAB Function/5(u_last)
  y2_derivative_sampling/1 -> MATLAB Function/2(y2_derivative_sampling)

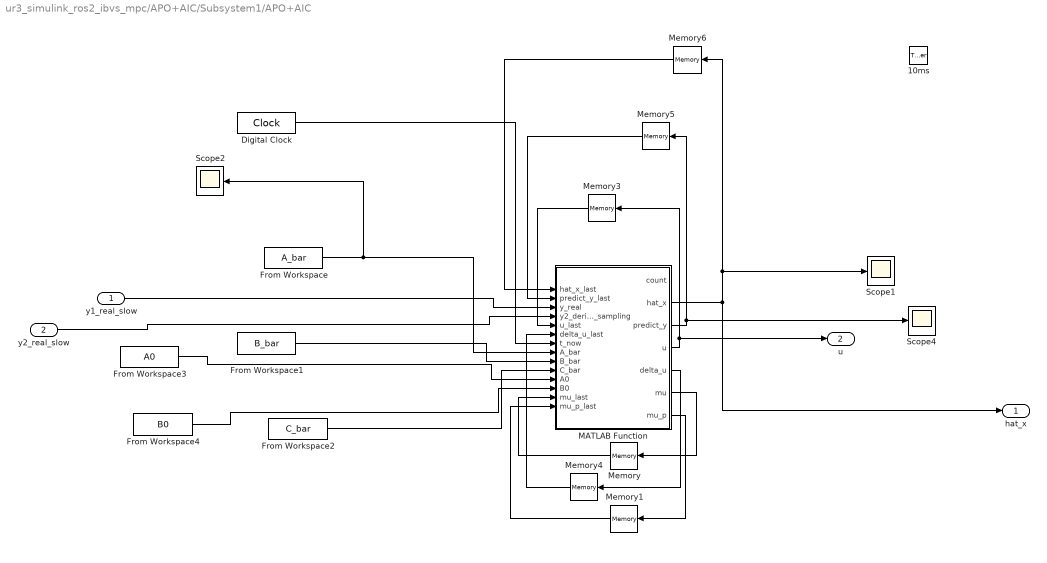
== system ur3_simulink_ros2_ibvs_mpc/APO+AIC/Subsystem1/APO+AIC ==
  y1_real_slow : Inport
  y2_real_slow : Inport  Port=2
  10ms : TriggerPort  VariantControl=(inherit)  InitialTriggerSignalState=zero  PortDimensions=1
  Digital Clock : DigitalClock  SampleTime=-1
  From Workspace : FromWorkspace  VariableName=A_bar  OutDataTypeStr=double  SampleTime=-1  OutputAfterFinalValue=Holding final value
  From Workspace1 : FromWorkspace  VariableName=B_bar  OutDataTypeStr=double  SampleTime=-1  OutputAfterFinalValue=Holding final value
  From Workspace2 : FromWorkspace  VariableName=C_bar  OutDataTypeStr=double  SampleTime=-1  OutputAfterFinalValue=Holding final value
  From Workspace3 : FromWorkspace  VariableName=A0  OutDataTypeStr=double  SampleTime=-1  OutputAfterFinalValue=Holding final value
  From Workspace4 : FromWorkspace  VariableName=B0  OutDataTypeStr=double  SampleTime=-1  OutputAfterFinalValue=Holding final value
  MATLAB Function : MATLAB Function  TreatAsAtomicUnit=on
  Memory{,1,3..6} (6 alike) : Memory  InheritSampleTime=on
  Scope1 : Scope
  Scope2 : Scope
  Scope4 : Scope
  hat_x : Outport
  u : Outport  Port=2
  wires:
  From Workspace2/1 -> MATLAB Function/10(C_bar)
  From Workspace1/1 -> MATLAB Function/9(B_bar)
  Digital Clock/1 -> MATLAB Function/7(t_now)
  Memory5/1 -> MATLAB Function/2(predict_y_last)
  MATLAB Function/3(predict_y) -> Memory5/1, Scope4/1
  From Workspace/1 -> Scope2/1, MATLAB Function/8(A_bar)
  MATLAB Function/2(hat_x) -> Memory6/1, Scope1/1, hat_x/1
  y1_real_slow/1 -> MATLAB Function/3(y_real)
  From Workspace3/1 -> MATLAB Function/11(A0)
  From Workspace4/1 -> MATLAB Function/12(B0)
  MATLAB Function/6(mu) -> Memory/1
  Memory/1 -> MATLAB Function/13(mu_last)
  MATLAB Function/7(mu_p) -> Memory1/1
  Memory1/1 -> MATLAB Function/14(mu_p_last)
  y2_real_slow/1 -> MATLAB Function/4(y2_derivative_sampling)
  MATLAB Function/4(u) -> Memory3/1, u/1
  Memory3/1 -> MATLAB Function/5(u_last)
  MATLAB Function/5(delta_u) -> Memory4/1
  Memory4/1 -> MATLAB Function/6(delta_u_last)
  Memory6/1 -> MATLAB Function/1(hat_x_last)

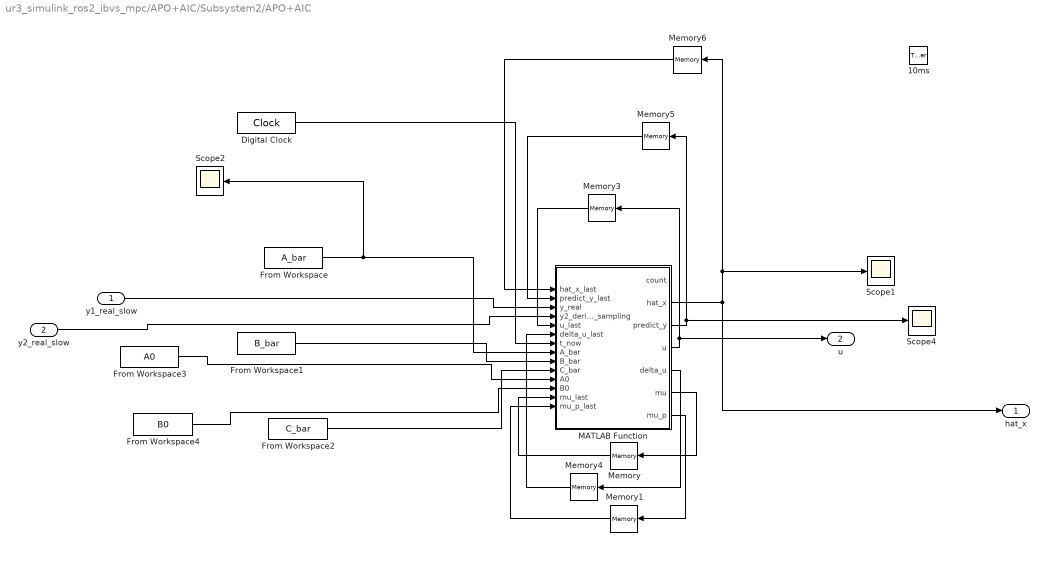
== system ur3_simulink_ros2_ibvs_mpc/APO+AIC/Subsystem2/APO+AIC ==
  y1_real_slow : Inport
  y2_real_slow : Inport  Port=2
  10ms : TriggerPort  VariantControl=(inherit)  InitialTriggerSignalState=zero  PortDimensions=1
  Digital Clock : DigitalClock  SampleTime=-1
  From Workspace : FromWorkspace  VariableName=A_bar  OutDataTypeStr=double  SampleTime=-1  OutputAfterFinalValue=Holding final value
  From Workspace1 : FromWorkspace  VariableName=B_bar  OutDataTypeStr=double  SampleTime=-1  OutputAfterFinalValue=Holding final value
  From Workspace2 : FromWorkspace  VariableName=C_bar  OutDataTypeStr=double  SampleTime=-1  OutputAfterFinalValue=Holding final value
  From Workspace3 : FromWorkspace  VariableName=A0  OutDataTypeStr=double  SampleTime=-1  OutputAfterFinalValue=Holding final value
  From Workspace4 : FromWorkspace  VariableName=B0  OutDataTypeStr=double  SampleTime=-1  OutputAfterFinalValue=Holding final value
  MATLAB Function : MATLAB Function  TreatAsAtomicUnit=on
  Memory{,1,3..6} (6 alike) : Memory  InheritSampleTime=on
  Scope1 : Scope
  Scope2 : Scope
  Scope4 : Scope
  hat_x : Outport
  u : Outport  Port=2
  wires:
  From Workspace2/1 -> MATLAB Function/10(C_bar)
  From Workspace1/1 -> MATLAB Function/9(B_bar)
  Digital Clock/1 -> MATLAB Function/7(t_now)
  Memory5/1 -> MATLAB Function/2(predict_y_last)
  MATLAB Function/3(predict_y) -> Memory5/1, Scope4/1
  From Workspace/1 -> Scope2/1, MATLAB Function/8(A_bar)
  MATLAB Function/2(hat_x) -> Memory6/1, Scope1/1, hat_x/1
  y1_real_slow/1 -> MATLAB Function/3(y_real)
  From Workspace3/1 -> MATLAB Function/11(A0)
  From Workspace4/1 -> MATLAB Function/12(B0)
  MATLAB Function/6(mu) -> Memory/1
  Memory/1 -> MATLAB Function/13(mu_last)
  MATLAB Function/7(mu_p) -> Memory1/1
  Memory1/1 -> MATLAB Function/14(mu_p_last)
  y2_real_slow/1 -> MATLAB Function/4(y2_derivative_sampling)
  MATLAB Function/4(u) -> Memory3/1, u/1
  Memory3/1 -> MATLAB Function/5(u_last)
  MATLAB Function/5(delta_u) -> Memory4/1
  Memory4/1 -> MATLAB Function/6(delta_u_last)
  Memory6/1 -> MATLAB Function/1(hat_x_last)

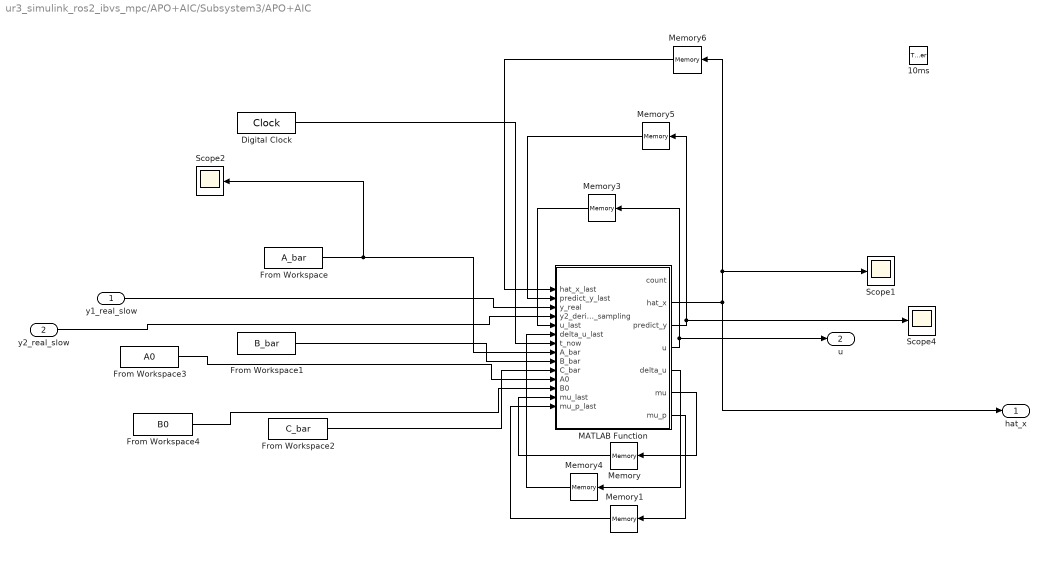
== system ur3_simulink_ros2_ibvs_mpc/APO+AIC/Subsystem3/APO+AIC ==
  y1_real_slow : Inport
  y2_real_slow : Inport  Port=2
  10ms : TriggerPort  VariantControl=(inherit)  InitialTriggerSignalState=zero  PortDimensions=1
  Digital Clock : DigitalClock  SampleTime=-1
  From Workspace : FromWorkspace  VariableName=A_bar  OutDataTypeStr=double  SampleTime=-1  OutputAfterFinalValue=Holding final value
  From Workspace1 : FromWorkspace  VariableName=B_bar  OutDataTypeStr=double  SampleTime=-1  OutputAfterFinalValue=Holding final value
  From Workspace2 : FromWorkspace  VariableName=C_bar  OutDataTypeStr=double  SampleTime=-1  OutputAfterFinalValue=Holding final value
  From Workspace3 : FromWorkspace  VariableName=A0  OutDataTypeStr=double  SampleTime=-1  OutputAfterFinalValue=Holding final value
  From Workspace4 : FromWorkspace  VariableName=B0  OutDataTypeStr=double  SampleTime=-1  OutputAfterFinalValue=Holding final value
  MATLAB Function : MATLAB Function  TreatAsAtomicUnit=on
  Memory{,1,3..6} (6 alike) : Memory  InheritSampleTime=on
  Scope1 : Scope
  Scope2 : Scope
  Scope4 : Scope
  hat_x : Outport
  u : Outport  Port=2
  wires:
  From Workspace2/1 -> MATLAB Function/10(C_bar)
  From Workspace1/1 -> MATLAB Function/9(B_bar)
  Digital Clock/1 -> MATLAB Function/7(t_now)
  Memory5/1 -> MATLAB Function/2(predict_y_last)
  MATLAB Function/3(predict_y) -> Memory5/1, Scope4/1
  From Workspace/1 -> Scope2/1, MATLAB Function/8(A_bar)
  MATLAB Function/2(hat_x) -> Memory6/1, Scope1/1, hat_x/1
  y1_real_slow/1 -> MATLAB Function/3(y_real)
  From Workspace3/1 -> MATLAB Function/11(A0)
  From Workspace4/1 -> MATLAB Function/12(B0)
  MATLAB Function/6(mu) -> Memory/1
  Memory/1 -> MATLAB Function/13(mu_last)
  MATLAB Function/7(mu_p) -> Memory1/1
  Memory1/1 -> MATLAB Function/14(mu_p_last)
  y2_real_slow/1 -> MATLAB Function/4(y2_derivative_sampling)
  MATLAB Function/4(u) -> Memory3/1, u/1
  Memory3/1 -> MATLAB Function/5(u_last)
  MATLAB Function/5(delta_u) -> Memory4/1
  Memory4/1 -> MATLAB Function/6(delta_u_last)
  Memory6/1 -> MATLAB Function/1(hat_x_last)

== system ur3_simulink_ros2_ibvs_mpc/Subsystem4/model refresher/get u and d ==
  u : Inport
  d : Inport  Port=2
  Bus Creator2 : BusCreator  Inputs=17
  MATLAB Function5 : MATLAB Function  TreatAsAtomicUnit=on
  U_in : Outport
  wires:
  MATLAB Function5/3(u3) -> Bus Creator2/3
  MATLAB Function5/1(u1) -> Bus Creator2/1
  MATLAB Function5/11(du3) -> Bus Creator2/11
  MATLAB Function5/8(dv1) -> Bus Creator2/8
  MATLAB Function5/12(dv3) -> Bus Creator2/12
  MATLAB Function5/9(du2) -> Bus Creator2/9
  MATLAB Function5/13(du4) -> Bus Creator2/13
  MATLAB Function5/14(dv4) -> Bus Creator2/14
  MATLAB Function5/6(u6) -> Bus Creator2/6
  MATLAB Function5/4(u4) -> Bus Creator2/4
  MATLAB Function5/5(u5) -> Bus Creator2/5
  MATLAB Function5/7(du1) -> Bus Creator2/7
  MATLAB Function5/2(u2) -> Bus Creator2/2
  MATLAB Function5/10(dv2) -> Bus Creator2/10
  u/1 -> MATLAB Function5/1(u)
  Bus Creator2/1 -> U_in/1
  d/1 -> MATLAB Function5/2(d)
  MATLAB Function5/15(dee_px) -> Bus Creator2/15
  MATLAB Function5/16(dee_py) -> Bus Creator2/16
  MATLAB Function5/17(dee_pz) -> Bus Creator2/17

== system ur3_simulink_ros2_ibvs_mpc/Subsystem5/attitude_pi_ctrl/Subsystem ==
  R_current : Inport
  Ts : Inport  Port=2
  Delay : Delay  DelayLength=1
  MATLAB Function : MATLAB Function  TreatAsAtomicUnit=on
  u : Outport
  wires:
  Ts/1 -> MATLAB Function/2(Ts)
  Delay/1 -> MATLAB Function/3(integral_error_last)
  MATLAB Function/1(u) -> u/1
  R_current/1 -> MATLAB Function/1(R_current)
  MATLAB Function/2(integral_error) -> Delay/1

== matlab function ur3_simulink_ros2_ibvs_mpc/Subsystem4/ref to square ==
  data: u input; y output size=[11,1]
function y = fcn(u)
y = zeros(11,1);
y(1) = u;
y(2) = u;
y(3) = u;
y(4) = -u;
y(5) = -u;
y(6) = -u;
y(7) = -u;
y(8) = u;
y(9) = 0;
y(10) = 0;
y(11) = 0;

== matlab function ur3_simulink_ros2_ibvs_mpc/joint vel to ros2/to ros2 ==
  data: u input; y output
function y  = fcn(u)
y = zeros(128,1);
y(1) = u(1);
y(2) = u(2);
y(3) = u(3);
y(4) = u(4);
y(5) = u(5);
y(6) = u(6);

== matlab function ur3_simulink_ros2_ibvs_mpc/MATLAB Function2 ==
  data: u input; y output
function y = fcn(u)
y = u(1:8);

== matlab function ur3_simulink_ros2_ibvs_mpc/Subsystem5/attitude_pi_ctrl/Subsystem/MATLAB Function ==
  data: R_current input; u output; Ts input; integral_error_last input; integral_error output
function [u,integral_error] = attitudePIDControl(R_current, Ts, integral_error_last)
    % 计算姿态误差矩阵
    Kp=-1;
    Ki=0;
    persistent R_target isFirstCall

    % 在第一次调用时初始化
    if isempty(isFirstCall)
        isFirstCall = false;
        R_target = R_current;  % 将当前姿态设置为目标姿态
    end
    % R_error = R_current * R_target';
    % 
    % % 计算旋转角度
    % theta = acos((trace(R_error) - 1) / 2);
    % 
    % % 计算旋转轴
    % if sin(theta) ~= 0
    %     v = 1 / (2*sin(theta)) * [R_error(3,2) - R_error(2,3); R_error(1,3) - R_error(3,1); R_error(2,1) - R_error(1,2)];
    % else
    %     v = [0; 0; 0]; % 对于非旋转的情况
    % end
    % 
    % % 误差向量
    % e = theta * v;
    % 
    % % PID控制器
    % % 比例项
    % P = Kp .* e;
    % 
    % % 积分项
    % integral_error = integral_error_last + e * Ts;
    % I = Ki .* integral_error;
    % 
    % % 控制信号
    % u = P + I;
    % u = R_current*u;


    % R_error = compute_qe(R_current, R_target);
    % qe_vec = R_error(2:4);
    % 
    % P = Kp .* qe_vec;
    % 
    % % 积分项
    % integral_error = integral_error_last + qe_vec .* Ts;
    % I = Ki * integral_error;
    % 
    % % 控制信号
    % u = P + I;
    % u = quat2rotm(R_current)' *u;

    R_error = R_target' * R_current - R_current' * R_target;
    e_R=[-R_error(2,3); R_error(1,3); R_error(2,1)];
    P = Kp .* e_R;

    % 积分项
    integral_error = integral_error_last + e_R * Ts;
    I = Ki .* integral_error;

    % 控制信号
    u = P + I;
    u = R_current*u;
end

% function qe = compute_qe(q, qd)
%     % Extract scalar (real) and vector (imaginary) parts
%     q0 = q(1);
%     q_vec = q(2:4);
%     q_vec=q_vec';
%     qd0 = qd(1);
%     qd_vec = qd(2:4);
%     qd_vec=qd_vec';
% 
%     % Calculate qe based on the provided equations
%     qe_vec = qd0 * q_vec - q0 * qd_vec + cross(q_vec, qd_vec);
%     qe0 = qd0 * q0 + qd_vec'* q_vec;
% 
%     % Combine the scalar and vector parts
%     qe = [qe0; qe_vec];
% end

== matlab function ur3_simulink_ros2_ibvs_mpc/Subsystem4/model refresher/get u and d/MATLAB Function5 ==
  data: u input; u1 output; u2 output; u3 output; u4 output; u5 output; u6 output; du1 output; dv1 output; du2 output; dv2 output; du3 output; dv3 output; du4 output; dv4 output; d input; dee_px output; dee_py output; dee_pz output
function [u1,u2,u3,u4,u5,u6,du1,dv1,du2,dv2,du3,dv3,du4,dv4,dee_px,dee_py,dee_pz] = fcn(u,d)
u1 = u(1);
u2 = u(2);
u3 = u(3);
u4 = u(4);
u5 = u(5);
u6 = u(6);
%disturbance
du1 = d(1);
dv1 = d(2);
du2 = d(3);
dv2 = d(4);
du3 = d(5);
dv3 = d(6);
du4 = d(7);
dv4 = d(8);
dee_px = d(9);
dee_py = d(10);
dee_pz = d(11);

== matlab function ur3_simulink_ros2_ibvs_mpc/Subsystem4/model refresher/to joint velocity ==
  data: new_jacobian output; ee_jacobian input; ee_rot input
function new_jacobian  = fcn(ee_jacobian, ee_rot)
rot_mat = [ee_rot,zeros(3,3);zeros(3,3),ee_rot];
new_jacobian = rot_mat*ee_jacobian;

== matlab function ur3_simulink_ros2_ibvs_mpc/APO+AIC/Subsystem1/APO+AIC/MATLAB Function ==
  data: count output; hat_x_last input; predict_y_last input; y_real input; y2_derivative_sampling input; u_last input; delta_u_last input; hat_x output; t_now input; A_bar input; B_bar input; C_bar input; predict_y output; A0 input; B0 input; mu_last input; mu_p_last input; u output; delta_u output; mu output; mu_p output
function [count,hat_x,predict_y, u, delta_u, mu, mu_p] = fcn(hat_x_last, predict_y_last, y_real,y2_derivative_sampling, u_last,delta_u_last,t_now,A_bar,B_bar,C_bar,A0,B0,mu_last, mu_p_last)
if(t_now==0)
    count=0;
    hat_x = zeros(2,1);
    predict_y = y_real;
    hat_x(1,1)=y_real;
    [u, delta_u, mu, mu_p]  = AIC2(t_now, 1, y_real,hat_x(1,1),y2_derivative_sampling,hat_x(2,1), mu_last, mu_p_last, u_last);
else
    count=mod(t_now,0.05);
    if(count==0)%在采样的时刻
        predict_y=y_real;
        hat_x=A_bar*hat_x_last +B_bar*delta_u_last/0.01+ C_bar*predict_y;
        [u, delta_u, mu, mu_p]  = AIC2(t_now, 1, y_real,hat_x(1,1),y2_derivative_sampling,hat_x(2,1), mu_last, mu_p_last, u_last);
    else%在两个采样时刻之间
        predict_y=[1 0]*(A0*hat_x_last+B0*delta_u_last);
        hat_x=A_bar*hat_x_last + B_bar*delta_u_last/0.01+C_bar*predict_y_last;
        [u, delta_u, mu, mu_p]  = AIC2(t_now, 1, y_real,hat_x(1,1),y2_derivative_sampling,hat_x(2,1), mu_last, mu_p_last, u_last);
    end
end
end








% function [count,hat_x,predict_y, u, delta_u, mu, mu_p, mu_pp] = fcn(hat_x_last, predict_y_last, y_real,y2_derivative_sampling,y3_real_slow, u_last,delta_u_last,t_now,A_bar,B_bar,C_bar,A0,B0,mu_last, mu_p_last, mu_pp_last)
% if(t_now==0)
%     count=0;
%     hat_x = zeros(3,1);
%     predict_y = y_real;
%     hat_x(1,1)=y_real;
%     u_now=0;
%     hat_x = A_bar*hat_x + B_bar*u_now+ C_bar*predict_y;
%     [u, delta_u, mu, mu_p, mu_pp]  = AIC3(t_now, 1, y_real,hat_x(1,1),y2_derivative_sampling,hat_x(2,1), y3_real_slow, hat_x(3,1), mu_last, mu_p_last, mu_pp_last, u_last);
%     %predict_y=[1 0 0]*(A0*hat_x+B0*delta_u); 
%     
% else
%     count=mod(t_now,0.05);
%     if(count==0)%在采样的时刻
%         predict_y=y_real;
%         hat_x=A_bar*hat_x_last +B_bar*delta_u_last+ C_bar*predict_y;
%         %hat_x(1,1)=y_real;
%         [u, delta_u, mu, mu_p, mu_pp]  = AIC3(t_now, 1, y_real,hat_x(1,1),y2_derivative_sampling,hat_x(2,1), y3_real_slow, hat_x(3,1), mu_last, mu_p_last, mu_pp_last, u_last);
% 
%         %predict_y=[1 0 0]*(A0*hat_x+B0*delta_u);
%         
%     else%在两个采样时刻之间
%         predict_y=[1 0 0]*(A0*hat_x_last+B0*delta_u_last);
%         hat_x=A_bar*hat_x_last + B_bar*delta_u_last+C_bar*predict_y_last;
%         [u, delta_u, mu, mu_p, mu_pp]  = AIC3(t_now, 1, y_real,hat_x(1,1),y2_derivative_sampling,hat_x(2,1), y3_real_slow, hat_x(3,1), mu_last, mu_p_last, mu_pp_last, u_last);
%         %predict_y=[1 0 0]*(A0*hat_x+B0*delta_u);
%         
%     end
% end
% end

== matlab function ur3_simulink_ros2_ibvs_mpc/norm jacobian ==
  data: u input; y output size=[6,6]
function y = fcn(u)
firstThreeColumns =u(1:3, :);
lastThreeColumns = u(4:6, :);
y = [lastThreeColumns;firstThreeColumns];

== matlab function ur3_simulink_ros2_ibvs_mpc/Subsystem3/MATLAB Function ==
  data: u input; joint1_pos output; joint2_pos output; joint3_pos output; joint4_pos output; joint5_pos output; joint6_pos output
function [joint1_pos,joint2_pos,joint3_pos,joint4_pos,joint5_pos,joint6_pos] = fcn(u)
joint1_pos = u(1);
joint2_pos = u(2);
joint3_pos = u(3);
joint4_pos = u(4);
joint5_pos = u(5);
joint6_pos = u(6);

== matlab function ur3_simulink_ros2_ibvs_mpc/APO+AIC/Subsystem2/APO+AIC/MATLAB Function ==
  data: count output; hat_x_last input; predict_y_last input; y_real input; y2_derivative_sampling input; u_last input; delta_u_last input; hat_x output; t_now input; A_bar input; B_bar input; C_bar input; predict_y output; A0 input; B0 input; mu_last input; mu_p_last input; u output; delta_u output; mu output; mu_p output
function [count,hat_x,predict_y, u, delta_u, mu, mu_p] = fcn(hat_x_last, predict_y_last, y_real,y2_derivative_sampling, u_last,delta_u_last,t_now,A_bar,B_bar,C_bar,A0,B0,mu_last, mu_p_last)
if(t_now==0)
    count=0;
    hat_x = zeros(2,1);
    predict_y = y_real;
    hat_x(1,1)=y_real;
    [u, delta_u, mu, mu_p]  = AIC2(t_now, 1, y_real,hat_x(1,1),y2_derivative_sampling,hat_x(2,1), mu_last, mu_p_last, u_last);
else
    count=mod(t_now,0.05);
    if(count==0)%在采样的时刻
        predict_y=y_real;
        hat_x=A_bar*hat_x_last +B_bar*delta_u_last/0.01+ C_bar*predict_y;
        [u, delta_u, mu, mu_p]  = AIC2(t_now, 1, y_real,hat_x(1,1),y2_derivative_sampling,hat_x(2,1), mu_last, mu_p_last, u_last);
    else%在两个采样时刻之间
        predict_y=[1 0]*(A0*hat_x_last+B0*delta_u_last);
        hat_x=A_bar*hat_x_last + B_bar*delta_u_last/0.01+C_bar*predict_y_last;
        [u, delta_u, mu, mu_p]  = AIC2(t_now, 1, y_real,hat_x(1,1),y2_derivative_sampling,hat_x(2,1), mu_last, mu_p_last, u_last);
    end
end
end








% function [count,hat_x,predict_y, u, delta_u, mu, mu_p, mu_pp] = fcn(hat_x_last, predict_y_last, y_real,y2_derivative_sampling,y3_real_slow, u_last,delta_u_last,t_now,A_bar,B_bar,C_bar,A0,B0,mu_last, mu_p_last, mu_pp_last)
% if(t_now==0)
%     count=0;
%     hat_x = zeros(3,1);
%     predict_y = y_real;
%     hat_x(1,1)=y_real;
%     u_now=0;
%     hat_x = A_bar*hat_x + B_bar*u_now+ C_bar*predict_y;
%     [u, delta_u, mu, mu_p, mu_pp]  = AIC3(t_now, 1, y_real,hat_x(1,1),y2_derivative_sampling,hat_x(2,1), y3_real_slow, hat_x(3,1), mu_last, mu_p_last, mu_pp_last, u_last);
%     %predict_y=[1 0 0]*(A0*hat_x+B0*delta_u); 
%     
% else
%     count=mod(t_now,0.05);
%     if(count==0)%在采样的时刻
%         predict_y=y_real;
%         hat_x=A_bar*hat_x_last +B_bar*delta_u_last+ C_bar*predict_y;
%         %hat_x(1,1)=y_real;
%         [u, delta_u, mu, mu_p, mu_pp]  = AIC3(t_now, 1, y_real,hat_x(1,1),y2_derivative_sampling,hat_x(2,1), y3_real_slow, hat_x(3,1), mu_last, mu_p_last, mu_pp_last, u_last);
% 
%         %predict_y=[1 0 0]*(A0*hat_x+B0*delta_u);
%         
%     else%在两个采样时刻之间
%         predict_y=[1 0 0]*(A0*hat_x_last+B0*delta_u_last);
%         hat_x=A_bar*hat_x_last + B_bar*delta_u_last+C_bar*predict_y_last;
%         [u, delta_u, mu, mu_p, mu_pp]  = AIC3(t_now, 1, y_real,hat_x(1,1),y2_derivative_sampling,hat_x(2,1), y3_real_slow, hat_x(3,1), mu_last, mu_p_last, mu_pp_last, u_last);
%         %predict_y=[1 0 0]*(A0*hat_x+B0*delta_u);
%         
%     end
% end
% end
